simulink model "RoutePlanner"  (R2023b)
settings: Solver=VariableStepAuto  StartTime=0.0  StopTime=1  RelTol=1e-3
undefined symbols (not defined in the file or in its folder): tsIntegrator
settings Model: Creator=cstabile  LastModifiedBy=cstabile
settings SFSimCC: SimTargetLang=C++

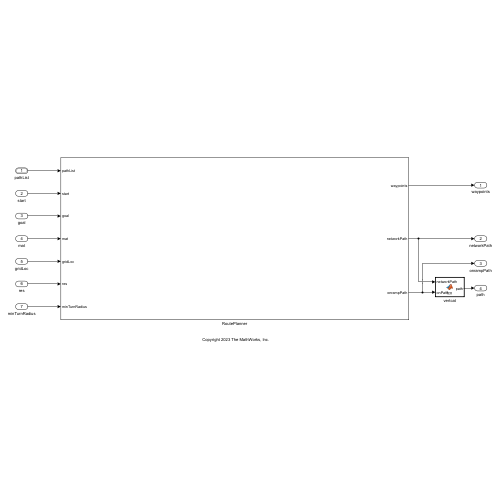
[thumbnail: Simulink's stored preview of the top-level diagram]
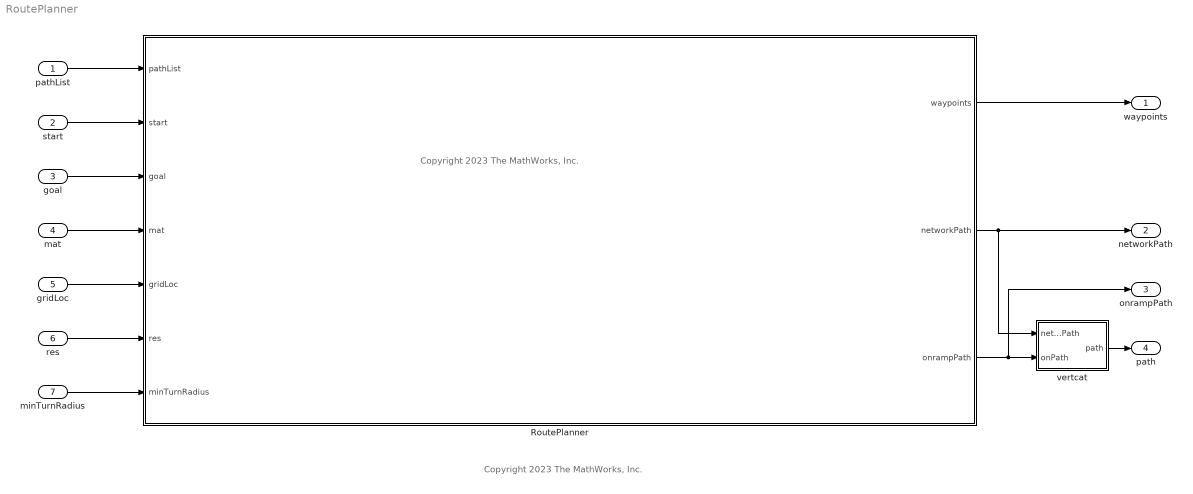
== system RoutePlanner ==
  note: Copyright 2023 The MathWorks, Inc.
  note: Copyright 2023 The MathWorks, Inc.
  pathList : Inport  OutDataTypeStr=Bus: pathList_fixed_bus  BusOutputAsStruct=on
  start : Inport  Port=2
  goal : Inport  Port=3
  mat : Inport  Port=4  OutDataTypeStr=boolean  PortDimensions=[1201 1201]
  gridLoc : Inport  Port=5  PortDimensions=[1 2]
  res : Inport  Port=6  PortDimensions=[1 1]
  minTurnRadius : Inport  Port=7
  RoutePlanner : Subsystem
  vertcat : MATLAB Function  TreatAsAtomicUnit=on
  waypoints : Outport  SampleTime=tsIntegrator
  networkPath : Outport  Port=2  SampleTime=tsIntegrator
  onrampPath : Outport  Port=3  SampleTime=tsIntegrator
  path : Outport  Port=4  SampleTime=tsIntegrator
  wires:
  mat/1 -> RoutePlanner/4(mat)
  RoutePlanner/2(networkPath) -> networkPath/1, vertcat/1(networkPath)
  goal/1 -> RoutePlanner/3(goal)
  RoutePlanner/1(waypoints) -> waypoints/1
  start/1 -> RoutePlanner/2(start)
  pathList/1 -> RoutePlanner/1(pathList)
  res/1 -> RoutePlanner/6(res)
  gridLoc/1 -> RoutePlanner/5(gridLoc)
  RoutePlanner/3(onrampPath) -> onrampPath/1, vertcat/2(onPath)
  vertcat/1(path) -> path/1
  minTurnRadius/1 -> RoutePlanner/7(minTurnRadius)

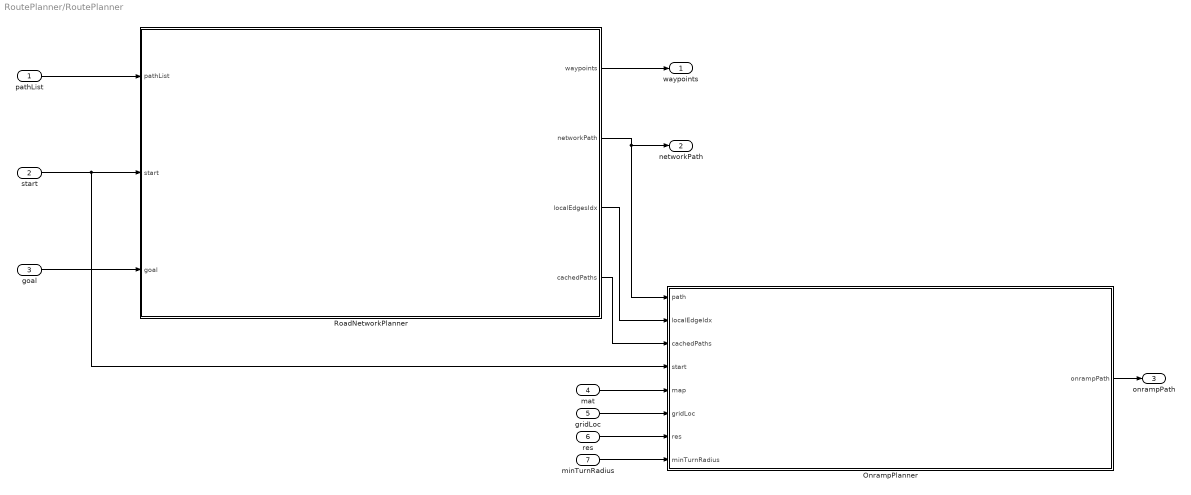
== system RoutePlanner/RoutePlanner ==
  pathList : Inport
  start : Inport  Port=2
  goal : Inport  Port=3
  mat : Inport  Port=4
  gridLoc : Inport  Port=5
  res : Inport  Port=6
  minTurnRadius : Inport  Port=7
  OnrampPlanner : Subsystem
  RoadNetworkPlanner : Subsystem
  waypoints : Outport
  networkPath : Outport  Port=2
  onrampPath : Outport  Port=3
  wires:
  mat/1 -> OnrampPlanner/5(map)
  goal/1 -> RoadNetworkPlanner/3(goal)
  pathList/1 -> RoadNetworkPlanner/1(pathList)
  RoadNetworkPlanner/1(waypoints) -> waypoints/1
  RoadNetworkPlanner/4(cachedPaths) -> OnrampPlanner/3(cachedPaths)
  RoadNetworkPlanner/3(localEdgesIdx) -> OnrampPlanner/2(localEdgeIdx)
  RoadNetworkPlanner/2(networkPath) -> OnrampPlanner/1(path), networkPath/1
  gridLoc/1 -> OnrampPlanner/6(gridLoc)
  res/1 -> OnrampPlanner/7(res)
  OnrampPlanner/1(onrampPath) -> onrampPath/1
  minTurnRadius/1 -> OnrampPlanner/8(minTurnRadius)
  start/1 -> OnrampPlanner/4(start), RoadNetworkPlanner/2(start)

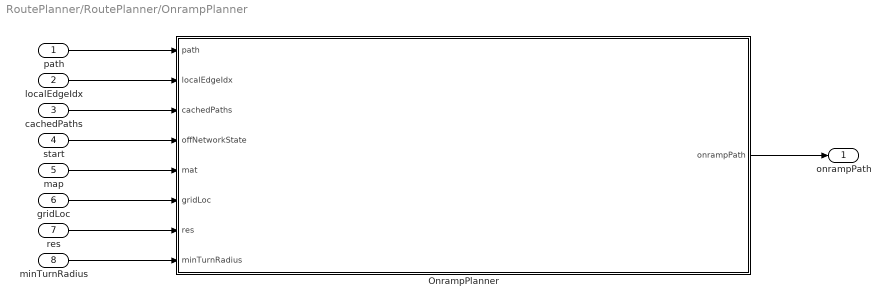
== system RoutePlanner/RoutePlanner/OnrampPlanner ==
  path : Inport
  localEdgeIdx : Inport  Port=2
  cachedPaths : Inport  Port=3
  start : Inport  Port=4
  map : Inport  Port=5
  gridLoc : Inport  Port=6
  res : Inport  Port=7
  minTurnRadius : Inport  Port=8
  OnrampPlanner : MATLAB Function  TreatAsAtomicUnit=on
  onrampPath : Outport
  wires:
  path/1 -> OnrampPlanner/1(path)
  start/1 -> OnrampPlanner/4(offNetworkState)
  OnrampPlanner/1(onrampPath) -> onrampPath/1
  map/1 -> OnrampPlanner/5(mat)
  localEdgeIdx/1 -> OnrampPlanner/2(localEdgeIdx)
  cachedPaths/1 -> OnrampPlanner/3(cachedPaths)
  gridLoc/1 -> OnrampPlanner/6(gridLoc)
  res/1 -> OnrampPlanner/7(res)
  minTurnRadius/1 -> OnrampPlanner/8(minTurnRadius)

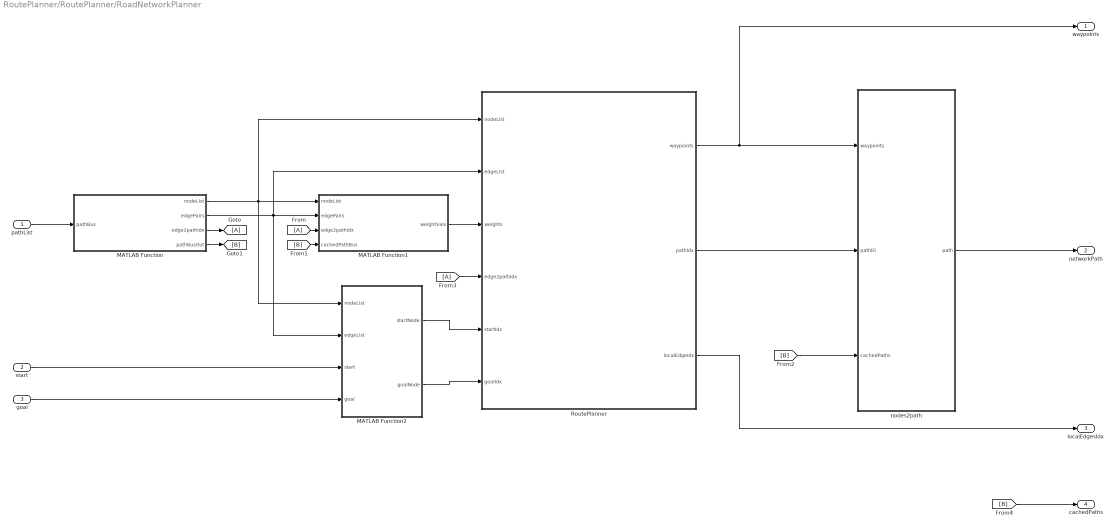
== system RoutePlanner/RoutePlanner/RoadNetworkPlanner ==
  pathList : Inport
  start : Inport  Port=2
  goal : Inport  Port=3  PortDimensions=[1 3]
  From : From
  From3 : From
  Goto : Goto
  MATLAB Function : MATLAB Function  TreatAsAtomicUnit=on  mask{maxElementPerEdge=inf, visualize=1}
      mask prompts: maxElementPerEdge "Max Path Elements Per Edge"; visualize "Visualize?"
  MATLAB Function1 : MATLAB Function  TreatAsAtomicUnit=on
  MATLAB Function2 : MATLAB Function  TreatAsAtomicUnit=on
  RoutePlanner : MATLAB Function  TreatAsAtomicUnit=on  mask{visualizeGraph=on}
      mask prompts: visualizeGraph "Visualize Graph?"
  nodes2path : MATLAB Function  TreatAsAtomicUnit=on
  waypoints : Outport
  networkPath : Outport  Port=2
  localEdgesIdx : Outport  Port=3
  cachedPaths : Outport  Port=4
  wires:
  MATLAB Function/2(edgePairs) -> MATLAB Function2/2(edgeList), MATLAB Function1/2(edgePairs), RoutePlanner/2(edgeList)
  MATLAB Function2/1(startNode) -> RoutePlanner/5(startIdx)
  MATLAB Function/1(nodeList) -> RoutePlanner/1(nodeList), MATLAB Function2/1(nodeList), MATLAB Function1/1(nodeList)
  RoutePlanner/1(waypoints) -> waypoints/1, nodes2path/1(waypoints)
  MATLAB Function/3(edge2pathIdx) -> Goto/1
  MATLAB Function1/1(weightVals) -> RoutePlanner/3(weights)
  MATLAB Function2/2(goalNode) -> RoutePlanner/6(goalIdx)
  MATLAB Function/4(pathBusOut) -> [B]
  RoutePlanner/2(pathIdx) -> nodes2path/2(pathID)
  [B] -> nodes2path/3(cachedPaths)
  From/1 -> MATLAB Function1/3(edge2pathIdx)
  [B] -> MATLAB Function1/4(cachedPathBus)
  start/1 -> MATLAB Function2/3(start)
  pathList/1 -> MATLAB Function/1(pathBus)
  goal/1 -> MATLAB Function2/4(goal)
  nodes2path/1(path) -> networkPath/1
  RoutePlanner/3(localEdgeIdx) -> localEdgesIdx/1
  From3/1 -> RoutePlanner/4(edge2pathIdx)
  [B] -> cachedPaths/1

== matlab function RoutePlanner/RoadNetworkPlanner/MATLAB Function ==
  data: pathBus input Bus: pathList_fixed_bus; nodeList output size=[inf 3]; edgePairs output size=[inf 2]; edge2pathIdx output size=[inf 1]; pathBusOut output Bus: pathList_variable_bus; maxElementPerEdge parameter; visualize parameter
function [nodeList,edgePairs,edge2pathIdx,pathBusOut] = paths2edges(pathBus,maxElementPerEdge,visualize)
    % Convert encoded bus to struct-array
    pathList = exampleHelperDecodeBus(pathBus);
    [nodeList,edgePairs,edge2pathIdx,cachedPaths] = exampleHelperPath2GraphData(pathList,maxElementPerEdge,visualize);

    % Convert list now containing duplicate/reverse edges to bus
    pathBusOut = exampleHelperEncodeBus(cachedPaths);
end

== matlab function RoutePlanner/RoadNetworkPlanner/RoutePlanner ==
  data: nodeList input; edgeList input; weights input; edge2pathIdx input; waypoints output size=[inf 2]; startIdx input; goalIdx input; pathIdx output size=[inf 1]; localEdgeIdx output size=[inf 1]; visualizeGraph parameter
function [waypoints, pathIdx, localEdgeIdx] = routePlanner(nodeList,edgeList,weights,edge2pathIdx,startIdx,goalIdx,visualizeGraph)
    persistent graphPlanner
    coder.extrinsic('exampleHelperVisualizeGraph');

    % Initialize graph if this is the first call
    if isempty(graphPlanner)
        stateTable = table(nodeList,VariableNames={'StateVector'});
        linkTable = table(edgeList, weights(:), edge2pathIdx(:), VariableNames={'EndStates','Weight','Edge2PathIdx'});
        graphPlanner = plannerAStar(navGraph(stateTable,linkTable));
    end

    % Plan a path on the graph
    [wps, solnInfo] = plan(graphPlanner,startIdx,goalIdx);
    waypoints = wps(:,1:2);

    % Convert network solution to path
    edgePairs = [solnInfo.PathStateIDs(1:end-1)' solnInfo.PathStateIDs(2:end)'];
    linkID = findlink(graphPlanner.Graph,edgePairs);
    pathIdx = graphPlanner.Graph.Links.Edge2PathIdx(linkID);

    % Retrieve all links connected to the initial node. These can be used
    % later to determine the path from initial state to network
    localSuccessors= successors(graphPlanner.Graph,solnInfo.PathStateIDs(1));
    localEdgeID = findlink(graphPlanner.Graph,[repelem(solnInfo.PathStateIDs(1),numel(localSuccessors),1) localSuccessors(:)]);

    % Return local edge list
    localEdgeIdx =  graphPlanner.Graph.Links.Edge2PathIdx(localEdgeID);

    if visualizeGraph
        exampleHelperVisualizeGraph(graphPlanner.Graph.States,graphPlanner.Graph.Links);
    end
end

== matlab function RoutePlanner/RoadNetworkPlanner/MATLAB Function1 ==
  data: nodeList input; edgePairs input; edge2pathIdx input; weightVals output size=[inf 1]; cachedPathBus input
function weightVals = computeEdgeWeights(nodeList, edgePairs, edge2pathIdx, cachedPathBus) %#ok<INUSD>
    persistent linkCosts

    if isempty(linkCosts)
        % Compute cost based on "euclidean" grid distance along path
        cachedPaths = exampleHelperDecodeBus(cachedPathBus);
        linkCosts = exampleHelperDefaultEdgeCost(cachedPaths,edge2pathIdx);
    end

    weightVals = linkCosts;
end

== matlab function RoutePlanner/RoadNetworkPlanner/MATLAB Function2 ==
  data: nodeList input; edgeList input; start input; startNode output; goal input; goalNode output
function [startNode,goalNode] = world2nearestnode(nodeList,edgeList,start,goal) %#ok<INUSD>
    [~,startNode] = min(vecnorm(nodeList(:,1:2)-start(1:2),2,2));
    [~,goalNode] = min(vecnorm(nodeList(:,1:2)-goal(1:2),2,2));
end

== matlab function RoutePlanner/RoadNetworkPlanner/nodes2path ==
  data: waypoints input; pathID input; cachedPaths input; path output size=[inf 3]
function path = nodesequence2smoothpath(waypoints, pathID, cachedPaths) %#ok<INUSD>
    % Convert network solution to path
    pathList = exampleHelperDecodeBus(cachedPaths);
    tmp = exampleHelperEncodeBus(pathList(pathID(:)));

    % Smooth path
    subsampleInterval = 3;
    path = exampleHelperSmoothPath(tmp.PointList,subsampleInterval);
end

== matlab function RoutePlanner/OnrampPlanner/OnrampPlanner ==
  data: path input; localEdgeIdx input; cachedPaths input; offNetworkState input size=[1 3]; onrampPath output size=[inf 3]; mat input; gridLoc input; res input; minTurnRadius input
function onrampPath = OnrampPlanner(path, localEdgeIdx, cachedPaths, offNetworkState, mat, gridLoc, res, minTurnRadius)
    localPathList = exampleHelperDecodeBus(cachedPaths);
    map = binaryOccupancyMap(mat,res);
    map.GridLocationInWorld = gridLoc(:)';
    onrampPath = exampleHelperConnectRSToPath(path, localPathList(localEdgeIdx), offNetworkState, map, minTurnRadius);
end

== matlab function RoutePlanner/vertcat ==
  data: networkPath input; path output; onPath input
function path = fcn(networkPath,onPath)

path = vertcat(onPath,networkPath);
